simulink model "bungee"  (R2018a)
settings: Solver=VariableStepAuto  StartTime=0.0  StopTime=50  RelTol=1e-3  EnableMultiTasking=on
PreLoadFcn:
  | % Execute script to load parameters
  | bungeeParams;
values from neighbouring files (symbols this model uses):
  A = 0.5    [bungeeParams.m]
  CD = 0.6    [bungeeParams.m]
  g = 9.81    [bungeeParams.m]
  k = 25    [bungeeParams.m]
  L = 20    [bungeeParams.m]
  m = 90    [bungeeParams.m]
  rho = 1.2    [bungeeParams.m]
  x0 = 80    [bungeeParams.m]
settings Model: Creator=nicholas  LastModifiedBy=bneiswan
settings DataIOCC: SaveFormat=Array  SaveState=on  SignalLoggingName=sigsOut
settings OptimizationCC: BlockReduction=off  BooleanDataType=off  ExpressionDepthLimit=2147483647  InitFltsAndDblsToZero=on  LifeSpan=inf
settings DebuggingCC: SaveWithParameterizedLinksMsg=none  UnderspecifiedInitializationDetection=Classic  MergeDetectMultiDrivingBlocksExec=none  CheckExecutionContextPreStartOutputMsg=on  CheckExecutionContextRuntimeOutputMsg=on  SignalResolutionControl=TryResolveAllWithWarning  MultiTaskDSMMsg=warning  MultiTaskCondExecSysMsg=none  ParameterPrecisionLossMsg=none  FcnCallInpInsideContextMsg=warning  AllowSymbolicDim=off  StateNameClashWarn=warning  SFUnexpectedBacktrackingDiag=warning  SFNoUnconditionalDefaultTransitionDiag=warning  SFExecutionAtInitializationDiag=none
settings HardwareCC: ProdBitPerPointer=32  ProdBitPerSizeT=32  ProdBitPerPtrDiffT=32  ProdLargestAtomicFloat=None  ProdIntDivRoundTo=Undefined  ProdEndianess=Unspecified  ProdWordSize=32  ProdHWDeviceType=32-bit Generic  TargetUnknown=on
settings ModelReferenceCC: PropagateSignalLabelsOutOfModel=off
settings CodeAppCC: StateflowObjectComments=on
settings GRTTargetCC: TargetFcnLib=ansi_tfl_tmw.mat  TargetLangStandard=C89/C90 (ANSI)  GeneratePreprocessorConditionals=Disable all  CombineOutputUpdateFcns=off  GRTInterface=on
settings ConfigComp: CovMetricSettings=dw  CovHtmlReporting=on  CovSaveCumulativeToWorkspaceVar=on  CovSaveSingleToWorkspaceVar=on  CovExternalEMLEnable=off  CovSFcnEnable=off

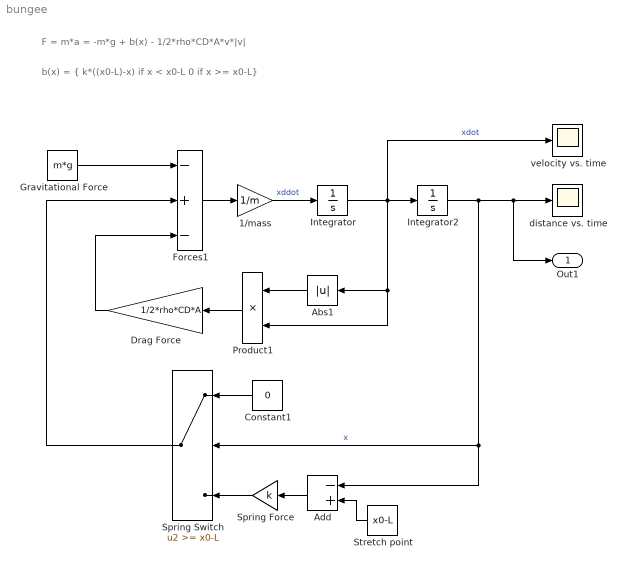
== system bungee ==
  note: b(x) = { k*((x0-L)-x) if x < x0-L
      | 0 if x >= x0-L}
  note: F = m*a = -m*g + b(x) - 1/2*rho*CD*A*v*|v|
  1/mass : Gain  Gain=1/m  SaturateOnIntegerOverflow=on  OutDataTypeStr=Inherit: Same as input  ParamDataTypeStr=Inherit: Same as input
  Abs1 : Abs
  Add : Sum  Inputs=-+
  Constant1 : Constant  Value=0
  Drag Force : Gain  Gain=1/2*rho*CD*A
  Forces1 : Sum  Inputs=-+-  SaturateOnIntegerOverflow=on  InputSameDT=on  OutDataTypeStr=Inherit: Same as first input
  Gravitational Force : Constant  Value=m*g
  Integrator : Integrator
      settings: AttributesFormatString=IC: %<InitialCondition>
  Integrator2 : Integrator  InitialCondition=x0
      settings: AttributesFormatString=IC: %<InitialCondition>
  Product1 : Product  RndMeth=Zero
  Spring Force : Gain  Gain=k  SaturateOnIntegerOverflow=on  OutDataTypeStr=Inherit: Same as input  ParamDataTypeStr=Inherit: Same as input
  Spring Switch : Switch  Threshold=x0-L  SaturateOnIntegerOverflow=on  InputSameDT=on
      settings: AttributesFormatString=Threshold = %<Threshold>
  Stretch point : Constant  Value=x0-L
  distance vs. time : Scope
  velocity vs. time : Scope
  Out1 : Outport
  wires:
  Spring Switch/1 -> Forces1/2
  Add/1 -> Spring Force/1
  1/mass/1 -> Integrator/1  "xddot"
  Integrator2/1 -> Out1/1, distance vs. time/1, Add/1, Spring Switch/2  "x"
  Abs1/1 -> Product1/1
  Constant1/1 -> Spring Switch/1
  Spring Force/1 -> Spring Switch/3
  Drag Force/1 -> Forces1/3
  Integrator/1 -> velocity vs. time/1, Integrator2/1, Abs1/1, Product1/2  "xdot"
  Forces1/1 -> 1/mass/1
  Product1/1 -> Drag Force/1
  Gravitational Force/1 -> Forces1/1
  Stretch point/1 -> Add/2
